simulink model "SimP"  (R2015a)
settings: Solver=ode45  StartTime=0.0  StopTime=60  RelTol=1e-3
settings Model: Creator=user  LastModifiedBy=user

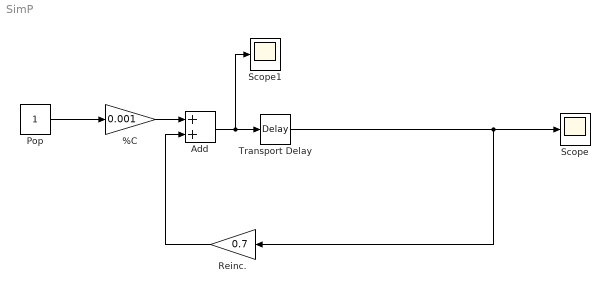
== system SimP ==
  %C : Gain  Gain=0.001
  Add : Sum
  Pop : Constant
  Reinc. : Gain  Gain=0.7
  Scope : Scope
  Scope1 : Scope
  Transport Delay : TransportDelay  DelayTime=8
  wires:
  %C/1 -> Add/1
  Transport Delay/1 -> Scope/1, Reinc./1
  Reinc./1 -> Add/2
  Add/1 -> Scope1/1, Transport Delay/1
  Pop/1 -> %C/1
